simulink subsystem "ForwardKinematicsRPM"  (R2024b)
settings: Solver=VariableStepAuto  StartTime=0.0  StopTime=10.0  RelTol=1e-3
undefined symbols (not defined in the file or in its folder): l, r
settings Model: Creator=Matthew  LastModifiedBy=Matthew

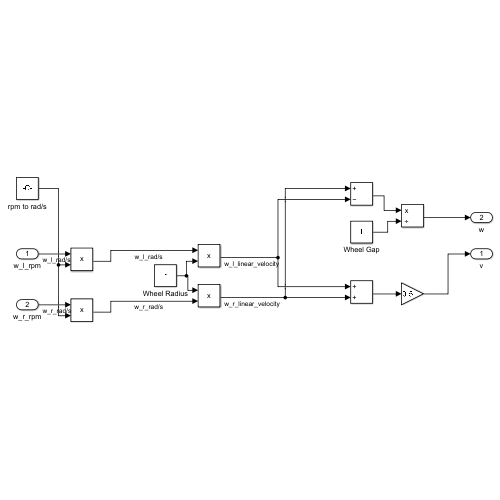
[thumbnail: Simulink's stored preview of the top-level diagram]
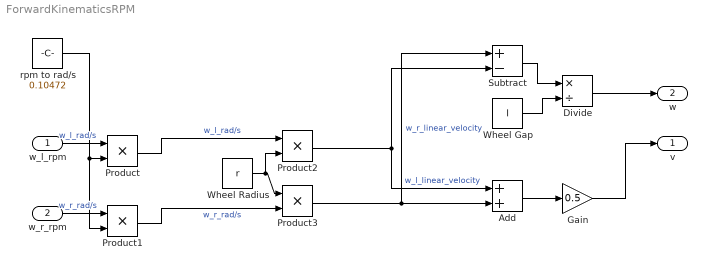
== system ForwardKinematicsRPM ==
  w_l_rpm : Inport
  w_r_rpm : Inport  Port=2
  Add : Sum
  Divide : Product  Inputs=*/
  Gain : Gain  Gain=0.5
  Product{,1..3} (4 alike) : Product
  Subtract : Sum  Inputs=+-
  Wheel Gap : Constant  Value=l
  Wheel Radius : Constant  Value=r
  rpm to rad/s : Constant  Value=0.10472
  v : Outport
  w : Outport  Port=2
  wires:
  Product/1 -> Product2/1  "w_l_rad/s"
  Product1/1 -> Product3/2  "w_r_rad/s"
  Subtract/1 -> Divide/1
  Wheel Gap/1 -> Divide/2
  Wheel Radius/1 -> Product2/2, Product3/1
  Product2/1 -> Subtract/2, Add/1  "w_l_linear_velocity"
  Product3/1 -> Add/2, Subtract/1  "w_r_linear_velocity"
  Divide/1 -> w/1
  Add/1 -> Gain/1
  Gain/1 -> v/1
  rpm to rad/s/1 -> Product1/2, Product/2
  w_r_rpm/1 -> Product1/1  "w_r_rad/s"
  w_l_rpm/1 -> Product/1  "w_l_rad/s"
